simulink model "TST_InnerTransition"  (Simulink 7.4)
settings: Solver=FixedStepDiscrete  StartTime=0.0  StopTime=10.0  FixedStep=0.02  RelTol=1e-3
settings Model: Creator=kharthforeign  LastModifiedBy=kharthforeign  BufferReuse=off
settings DataIOCC: SaveOutput=off  SignalLogging=off  SaveTime=off
settings OptimizationCC: BlockReduction=off  ConditionallyExecuteInputs=off  OptimizeBlockIOStorage=off  BufferReuse=off  ExpressionFolding=off  LocalBlockOutputs=off  InitFltsAndDblsToZero=on

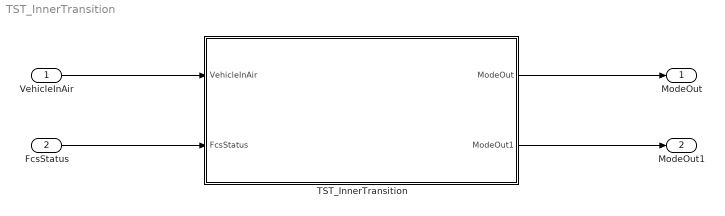
== system TST_InnerTransition ==
  VehicleInAir : Inport  PortDimensions=1  DataType=boolean  OutDataType=fixdt(1, 16)  OutScaling=2^0  OutDataTypeStr=boolean
  FcsStatus : Inport  Port=2  UseBusObject=on  OutDataType=fixdt(1, 16)  OutScaling=2^0
      settings: BusObject=FCS_FlightControlSystem_Status
  TST_InnerTransition : Subsystem  TreatAsAtomicUnit=on
  ModeOut : Outport  PortDimensions=1  DataType=uint32  OutDataType=Enum: GBL_Definitions_EjectionCmd  OutDataTypeStr=uint32
  ModeOut1 : Outport  Port=2  PortDimensions=1  DataType=uint32  OutDataType=Enum: GBL_Definitions_EjectionCmd  OutDataTypeStr=uint32
  wires:
  VehicleInAir/1 -> TST_InnerTransition/1(VehicleInAir)
  FcsStatus/1 -> TST_InnerTransition/2(FcsStatus)
  TST_InnerTransition/1(ModeOut) -> ModeOut/1
  TST_InnerTransition/2(ModeOut1) -> ModeOut1/1

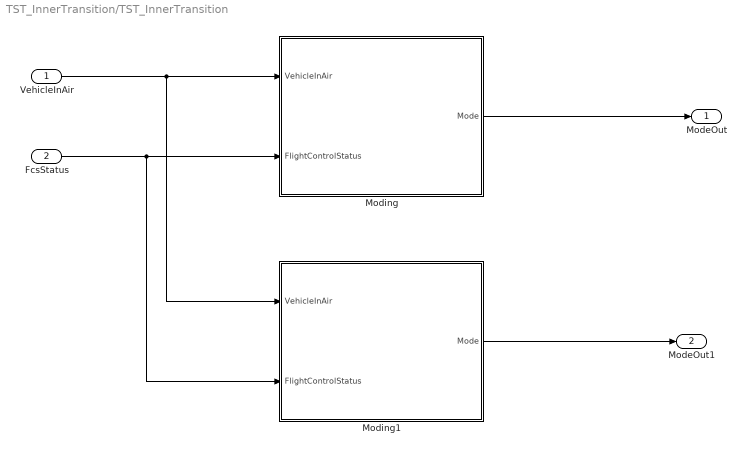
== system TST_InnerTransition/TST_InnerTransition ==
  VehicleInAir : Inport  PortDimensions=1  DataType=boolean  OutDataType=fixdt(1, 16)  OutScaling=2^0  OutDataTypeStr=boolean
  FcsStatus : Inport  Port=2  UseBusObject=on  OutDataType=fixdt(1, 16)  OutScaling=2^0
      settings: BusObject=FCS_FlightControlSystem_Status
  Moding : Stateflow chart  TreatAsAtomicUnit=on
  Moding1 : Stateflow chart  TreatAsAtomicUnit=on
  ModeOut : Outport  PortDimensions=1  DataType=uint32  OutDataType=Enum: GBL_Definitions_EjectionCmd  OutDataTypeStr=uint32
  ModeOut1 : Outport  Port=2  PortDimensions=1  DataType=uint32  OutDataType=Enum: GBL_Definitions_EjectionCmd  OutDataTypeStr=uint32
  wires:
  FcsStatus/1 -> Moding/2(FlightControlStatus), Moding1/2(FlightControlStatus)
  VehicleInAir/1 -> Moding/1(VehicleInAir), Moding1/1(VehicleInAir)
  Moding/1(Mode) -> ModeOut/1
  Moding1/1(Mode) -> ModeOut1/1

== stateflow chart TST_InnerTransition/Moding ==
  state Main
    state Off
      entry:
      Mode = uint32(1);
    state Launch
      entry:
      Mode = uint32(2);
    state Autoland
      entry:
      Mode = uint32(3);
    Main -> (junction 9) : [true]
    (junction 9) -> Off [order 1] : [(FlightControlStatus.PressureAltitude_Ft < 500.0) && (~VehicleInAir)]
    (junction 9) -> (junction 10) [order 2]
    (junction 10) -> Launch [order 1] : [(FlightControlStatus.PressureAltitude_Ft > 1500.0) || VehicleInAir]
    (junction 10) -> (junction 11) [order 2]
    (junction 11) -> Autoland : [(FlightControlStatus.PressureAltitude_Ft > 2500.0) || ...
        | FlightControlStatus.LeftEngFailed]
    (default) -> Off : {UpdateFeedthroughParameters();}
  state UpdateFeedthroughParameters [function]
    (default) -> (junction 8) : {...
        |    Mode = uint32(5);...
        | }
  (default) -> Main
  data: VehicleInAir input boolean; Mode output uint32; FlightControlStatus input FCS_FlightControlSystem_Status

== stateflow chart TST_InnerTransition/Moding1 ==
  state Main
    state Off
      entry:
      Mode = uint32(1);
    state Launch
      entry:
      Mode = uint32(2);
    state Autoland
      entry:
      Mode = uint32(3);
    (default) -> Off : {UpdateFeedthroughParameters();}
    Main -> Off [order 1] : [(FlightControlStatus.PressureAltitude_Ft < 500.0) && (~VehicleInAir)]
    Main -> Autoland [order 3] : [(FlightControlStatus.PressureAltitude_Ft > 2500.0) || ...
        | FlightControlStatus.LeftEngFailed]
    Main -> Launch [order 2] : [(FlightControlStatus.PressureAltitude_Ft > 1500.0) || VehicleInAir]
  state UpdateFeedthroughParameters [function]
    (default) -> (junction 31) : {...
        |    Mode = uint32(5);...
        | }
  (default) -> Main
  data: VehicleInAir input boolean; Mode output uint32; FlightControlStatus input FCS_FlightControlSystem_Status
